simulink model "regler_bsp"  (R2023a)
settings: Solver=VariableStepAuto  StartTime=0.0  StopTime=10.0  RelTol=1e-3
settings Model: Creator=berkayozgur  LastModifiedBy=berkayozgur

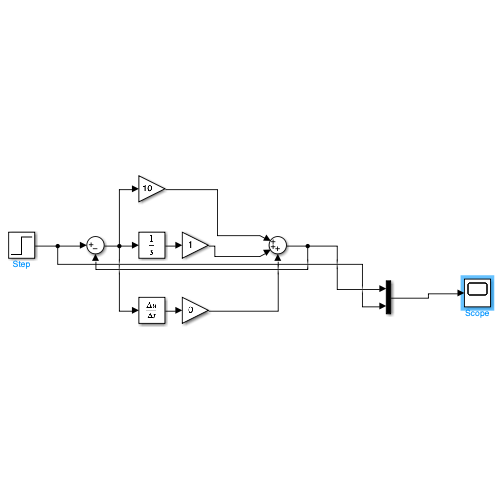
[thumbnail: Simulink's stored preview of the top-level diagram]
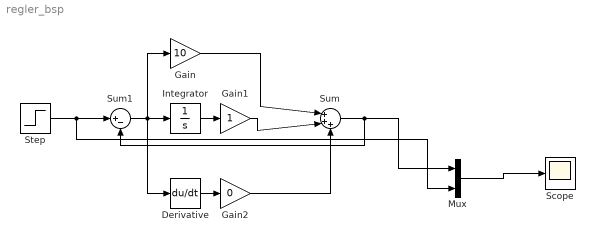
== system regler_bsp ==
  Derivative : Derivative
  Gain : Gain  Gain=10
  Gain1 : Gain
  Gain2 : Gain  Gain=0
  Integrator : Integrator
  Mux : Mux  Inputs=2
  Scope : Scope
  Step : Step  SampleTime=0
  Sum : Sum  Inputs=|+++
  Sum1 : Sum  Inputs=|+-
  wires:
  Gain/1 -> Sum/1
  Integrator/1 -> Gain1/1
  Derivative/1 -> Gain2/1
  Sum/1 -> Mux/1, Sum1/2
  Gain1/1 -> Sum/2
  Gain2/1 -> Sum/3
  Mux/1 -> Scope/1
  Step/1 -> Mux/2, Sum1/1
  Sum1/1 -> Derivative/1, Gain/1, Integrator/1
